simulink model "connecttoUDP_final"  (R2025a)
settings: Solver=ode4  StartTime=0.0  StopTime=inf  FixedStep=1/500  RelTol=1e-3  EnableMultiTasking=on
InitFcn:
  | home = [0.45; 0; 0.49];
  | pick = [0.3; 0; 0.3];
  | place = [-0.25; -0.25; 0.01];
  | waypoints = ...
  | [pick, pick,place ,place ,home]' ;
undefined symbols (not defined in the file): HIL, qc_get_step_size
libraries: quarc_library x19, simulink x3
(part 2 of 2)

== matlab function connecttoUDP_final/MATLAB Function ==
  settings: updateMethod=DISCRETE
  data: number output; p4 input; python_cmd input; gripper_cmd output; t input; is_visible input; gesto_to_int input; search_pos output
function [number, gripper_cmd, search_pos] = StateMachine(p4, python_cmd, t, is_visible, gesto_to_int)    
    
    persistent state
    persistent t_travel
    persistent t_visible
    persistent t_lost
    persistent t_gesture
    persistent current_y

    if isempty(state)
        state = 2; % 0 = Hunting the ball down, 1 = Going back to goal, 2 = Returning home and search
        t_travel = -1; % Putting a negative time stops the timer, used to find the travel time in each state mode
        t_visible = -1;
        t_lost = -1;
        t_gesture = -1;
        current_y = 0;
    end
    
    % Default safe position to output when not in State 2
    search_pos = [0.25; 0; 0.50];

    % --- Machine State Logic ---
    switch state
        
        case 0 % STATE 0: HUNTING THE BALL
            number = 1; % Connected on port 1 (xyz_mean)
            gripper_cmd = python_cmd; % The claw follows the camera
            
            % 1. CHECK IF BALL WAS CAUGHT
            if python_cmd == 1
                state = 3; 
                t_lost = -1; % Reset lost timer just in case
            end
            
            % 2. WATCHDOG TIMER: IF BALL IS LOST
            % If the camera goes blind, start the stopwatch before aborting
            if is_visible == 0
                if t_lost == -1
                    t_lost = t; % Start the lost stopwatch
                elseif (t - t_lost) >= 2.5 % Lost for more than 2.5 seconds
                    state = 2; % Go back to search mode
                    t_lost = -1; % Reset timer
                end
            else
                % Ball is visible, reset the stopwatch (Debounce)
                t_lost = -1; 
            end
            
        case 1 % STATE 1: DELIVERY (Advance in a straight line and release)
            number = 2; % We use port 2 to send a dynamic search_pos
            
            % 1. CALCULATE THE DYNAMIC TARGET POSITION
            % X was 0.25. We scale it by 2
            % Y is scaled by 2 in the exact same direction
            % Z is lowered to 0.40m
            target_x = 0.25 * 2; 
            target_y = current_y * 2;
            target_pos = [target_x; target_y; 0.40];
            
            % Send this position to the kinematics
            search_pos = target_pos; 
            
            % 2. IDENTIFY ARRIVAL AT TARGET
            distance_goal = norm(p4(1:3) - target_pos);
            
            if distance_goal < 0.05 && t_travel == -1
                t_travel = t; % Arrived! Start the delivery stopwatch  
            end
            
            % 3. DELIVERY TIMER LOGIC (Wait 1.0s -> Drop -> Wait 1s -> Leave)
            if t_travel ~= -1
                % If 4 seconds have passed (1.0s holding + 1s letting go)
                if (t - t_travel) >= 2.0
                    state = 2; % Mission accomplished! Return to Home/Search
                    t_travel = -1; % Reset timer
                    current_y = 0; % Reset joystick memory for next time
                    gripper_cmd = 1; % Claw still closed
                    
                % If 3 seconds have passed
                elseif (t - t_travel) >= 1.0 
                    gripper_cmd = 0; % OPEN CLAW (Drop the ball)
                    
                % If arrived but still waiting the initial 3 seconds
                else
                    gripper_cmd = 1; % KEEP CLAW CLOSED
                end
                
            else
                % Still traveling to the target
                gripper_cmd = 1; % Keep holding the ball tight
            end

        case 2 % STATE 2: SEARCH MODE (Go to alert position and sweep)
            number = 2; % Connected on port 2 (Search position)
            gripper_cmd = 0; % Keep claw open to not grab ghosts
            
            % 1. IDENTIFY ARRIVAL AT ALERT POSITION (Home)
            % Calculates distance to the base center position [0.25; 0; 0.50]
            distance_home = norm(p4(1:3) - [0.25; 0; 0.50]); 
            
            if distance_home < 0.05 && t_travel == -1
                t_travel = t; 
            end
            
            % 2. EXECUTE THE SINE WAVE SWEEP
            if t_travel == -1
                % Not there yet, keep target strictly at the center
                search_pos = [0.25; 0; 0.50];
            else
                % Start oscillating the Y axis                
                y_sweep = 0.25 * sin(0.30 * (t - t_travel));
                search_pos = [0.25; y_sweep; 0.50];
            end
            
            % 3. VERIFICATION BARRIER (DEBOUNCE LOGIC)
            if is_visible == 1
                if t_visible == -1
                    t_visible = t; % Ball spotted, start the stopwatch
                elseif (t - t_visible) >= 0.25 % Has it been consistently visible for 0.25 second
                    state = 0; % Barrier cleared! Transition to HUNTING
                    t_travel = -1; % Reset sweep timer
                    t_visible = -1; % Reset vision timer
                end
            else
                % False alarm or lost sight --> Reset stopwatch immediately
                t_visible = -1;
            end             

        case 3 % STATE 3: HOLD TARGET AND GESTURE JOYSTICK CONTROL
            number = 2; % Connect on port 2 (Search/Home position)
            gripper_cmd = 1; % KEEP CLAW CLOSED (Holding the ball)
            
            % 1. IDENTIFY ARRIVAL AT ALERT POSITION (Home)
            % Calculates distance to the base center position [0.25; 0; 0.50]
            distance_home = norm(p4(1:3) - [0.25; 0; 0.50]); 
            
            if distance_home < 0.05 && t_travel == -1
                t_travel = t; % Arrived! Unlock joystick control
                current_y = 0; % Reset joystick position to absolute center
            end
            
            % 2. EXECUTE THE JOYSTICK MOVEMENT BASED ON GESTURE
            if t_travel == -1
                % Not there yet, keep target strictly at the center
                search_pos = [0.25; 0; 0.50];
            else
                % Arrived at center. Now read the gesture to move!
                if gesto_to_int == 3 % RIGHT
                    current_y = current_y + 0.00010; % Move right smoothly
                    
                elseif gesto_to_int == 4 % LEFT
                    current_y = current_y - 0.00010; % Move left smoothly
                    
                end
                % Note: If gesture is NONE (0) or HAND (2), current_y is NOT modified. 
                % This creates the "freeze in place" smooth stop effect!
                
                % 3. SAFETY CLAMP (Mechanical Limits)
                % Prevent the arm from rotating beyond safe boundaries
                if current_y > 0.25
                    current_y = 0.25;
                elseif current_y < -0.25
                    current_y = -0.25;
                end
                
                % Output the accumulated position to the kinematics
                search_pos = [0.25; current_y; 0.50];
            end
            
            % 4. STOP GESTURE AND TRANSITION (With Debounce/Safety)
            % If the stop sign is shown AND the robot is already parked
            if gesto_to_int == 1 && t_travel ~= -1
                if t_gesture == -1
                    t_gesture = t; % AI saw STOP! Start the stopwatch
                elseif (t - t_gesture) >= 0.5 % Has it been a STOP for 0.5s?
                    state = 1; % Transition to the DELIVERY state
                    t_travel = -1; % Reset timer for the next state
                    t_gesture = -1; % Reset gesture timer
                end
            else
                % If it's not a STOP sign (false alarm or still moving), reset stopwatch
                t_gesture = -1; 
            end
            
        otherwise
            % Security against bugs 

            % 1. Fallback to the safest physical state
            state = 2; 
            number = 2; 
            search_pos = [0.25; 0; 0.50]; 
            gripper_cmd = 0; 
            
            % 2. Wipe all memory clean (Reset all timers)
            t_travel = -1;
            t_visible = -1;
            t_lost = -1;
            t_gesture = -1;
            current_y = 0;
    end
end

== matlab function connecttoUDP_final/TargetRangeLimiter ==
  data: p_obj_0 input; p_target output; R_max input
function p_target = radialClamp(p_obj_0, R_max)

eps_val = 1e-6;

norm_p = norm(p_obj_0);

if norm_p > R_max
    p_target = R_max * (p_obj_0 / (norm_p + eps_val));
else
    p_target = p_obj_0;
end

end

== matlab function connecttoUDP_final/MATLAB Function1 ==
  data: udp_data input size=[8 1]; t input size=1; X_filt output; Y_filt output; Z_filt output; gripper_cmd output; is_visible output; gesture_cmd output
function [X_filt, Y_filt, Z_filt, gripper_cmd, is_visible, gesture_cmd] = HybridSensorKalman(udp_data, t)
    % udp_data is a 7x1 vector from Python: 
    % [SensX, SensY, SensZ, PinhX, PinhY, PinhZ, FoundFlag]
    
    % Define the variables that will remember their values between Simulink steps
    persistent x_est P kf_initialized t_grip_start consecutive_outliers is_gripping

    % Initialize the Kalman Filter
    if isempty(kf_initialized)
        x_est = [0.2; 0.0; 0.3];  % Initial guess (Safe home position)
        P = eye(3) * 1.0;         % Initial uncertainty
        kf_initialized = true;
        t_grip_start = -1;        % Timer for gripper delay
        consecutive_outliers = 0; % Start counting outliers
        is_gripping = 0;          % Initialize grip state
    end

    % 1. Unpack UDP data and force double precision
    z_sens = double(udp_data(1:3));
    z_pinh = double(udp_data(4:6));
    found_flag = double(udp_data(7));
    gesture_cmd = double(udp_data(8));
    is_visible = found_flag;
    
    % Kalman tuning parameters (to be adjusted through trial and error)
    Q = eye(3) * 1e-6;   % Process Noise
    R_val = 8e-6;        % Measurement Variance

    % 2. Constant Position Kalman Prediction
    x_est = x_est;
    P = P + Q;

    % 3. Kalman Update (Sensor Fusion)
    if found_flag == 1
        % Determine depth
        depth = z_sens(3);
        if depth == 0 % Blind sensor scenario
            depth = z_pinh(3);
        end
        
        % Dynamic Confidence (Soft Switch)
        if depth < 0.25
            % Very close: Trust Pinhole 100%, Sensor 0%
            w_sens = 0.0; 
            w_pinh = 1.0;
        elseif depth > 0.35
            % Far away: Trust Sensor 100%, Pinhole 0%
            w_sens = 1.0; 
            w_pinh = 0.0;
        else
            % Transition Zone (25cm to 35cm): Cross-fade the signals
            w_sens = (depth - 0.25) / 0.10; 
            w_pinh = 1.0 - w_sens;
        end
        
        % Fused depth estimation
        z_fused = (w_sens * z_sens) + (w_pinh * z_pinh);
        
        % Outlier Detection (We check the Z depth specifically)
        distance_jump = abs(z_fused(3) - x_est(3));
        if distance_jump < 0.15
            % Normal Kalman update
            R = eye(3) * R_val;
            K = P / (P + R);
            x_est = x_est + K * (z_fused - x_est);
            P = (eye(3) - K) * P;

            consecutive_outliers = 0; % Reset counter

        else
            % Outlier detected
            consecutive_outliers = consecutive_outliers + 1;
            
            if consecutive_outliers > 3
                % Update position if not outlier
                x_est = z_fused;
                P = eye(3) * 1.0; % Reset uncertainty
                consecutive_outliers = 0;
            end
        end
    end

    % 4. Output filtered coordinates
    X_filt = x_est(1);
    Y_filt = x_est(2);
    Z_filt = x_est(3);

    % 5. Gripper Delay Logic
    dist_to_target = norm(x_est);

    if is_gripping == 0
        % Waiting for object
        if found_flag == 1 && dist_to_target <= 0.25
            if t_grip_start == -1
                t_grip_start = t; % Start timer
            elseif (t - t_grip_start) >= 0.75 
                is_gripping = 1; 
            end
        else
            t_grip_start = -1; % Reset timer if object moves away
        end
    else
        % Holding the object
        if gesture_cmd == 1
            is_gripping = 0;   % Release latch
            t_grip_start = -1; % Reset timer
        end
    end
    
    % Output the persistent state to the hardware
    gripper_cmd = is_gripping; 
end

== matlab function connecttoUDP_final/Champ cartésien ==
  data: p_current input; p_cmd output; p_target input; is_visible input
function  p_cmd= potentialFieldPlanner(p_current, p_target, is_visible)
% p_current : [3x1]
% p_target   : [3x1]
% is_visible: 0/1
% Ts        : pas de temps

%% Paramètres
k_att = 3.0;       % gain attractif
k_rep = 0.05;      % gain répulsif cylindre
v_max = 0.25;      % vitesse cartésienne max [m/s]

d0 = 0.15;         % rayon d'influence du cylindre
eps_norm = 1e-6;   % protection division par zéro

Ts=0.25

%% Si cible non visible : on garde la position actuelle
if is_visible == 0
    p_cmd = p_current;
    return;
end

%% --- Champ attractif ---
e = p_target - (p_current-[0.0;0.0;0.2]);
F_att = k_att * e;

%% --- Champ répulsif cylindre autour de la base ---
x = p_current(1);
y = p_current(2);
d = sqrt(x^2 + y^2);


if d < d0 && d > eps_norm
    n = [x; y; 0] / (d + eps_norm);
    F_rep = k_rep * (1/d - 1/d0) * (1/(d^2 + eps_norm)) * n;
else 
    F_rep=[0.0;0.0;0.0];
end

%% --- Champ total ---
F = F_att + F_rep;

%% --- Saturation smooth ---
F_norm = norm(F);

if F_norm > eps_norm
    v_cmd = v_max * tanh(F_norm / v_max) * (F / F_norm);
else
    v_cmd = [0;0;0];
end

%% --- Pas d'Euler ---
p_cmd = p_current + Ts * v_cmd;

end

== matlab function connecttoUDP_final/forward kinematics1 ==
  data: p3 output; R03 output; phi input; p4 output; R04 output; p_cam_0 output; p_obj_0 output; p_obj_cam input
function [p3, R03, p4, R04, p_cam_0,p_obj_0] = qarmForwardKinematics(phi,p_obj_cam)

%% QUANSER_ARM_FPK
% v 4.0 - 4th June 2020

% REFERENCE: 
% Chapter 3. Forward Kinematics
% Robot Dynamics and Control 
% Spong, Vidyasagar
% 1989

% INPUTS:
% phi     : Alternate joint angles vector 4 x 1

% OUTPUTS:
% p4      : End-effector frame {4} position vector expressed in base frame {0}
% R04     : rotation matrix from end-effector frame {4} to base frame {0}

%% Manipulator parameters:
L1 = 0.1400;
L2 = 0.3500;
L3 = 0.0500;
L4 = 0.2500;
L5 = 0.1500;

%% Alternate parameters
l1 = L1;
l2 = sqrt(L2^2 + L3^2);
l3 = L4 + L5;
beta = atan(L3/L2);

%% From phi space to theta space 
theta = phi;
theta(1) = phi(1);
theta(2) = phi(2) + beta - pi/2;
theta(3) = phi(3) - beta;
theta(4) = phi(4);

%% Transformation matrices for all frames:

% T{i-1}{i} = quanser_arm_DH(  a, alpha,  d,     theta );
        T01 = quanser_arm_DH(  0, -pi/2, l1,  theta(1) );
        T12 = quanser_arm_DH( l2,     0,  0,  theta(2) );
        T23 = quanser_arm_DH(  0, -pi/2,  0,  theta(3) );
        T34 = quanser_arm_DH(  0,     0, l3,  theta(4) );

        T02 = T01*T12;
        T03 = T02*T23;
        T04 = T03*T34;

%% Position of end-effector Transformation

% Extract the Position vector 
% p1   = T01(1:3,4);
% p2   = T02(1:3,4);
p3   = T03(1:3,4);
p4   = T04(1:3,4);

% Extract the Rotation matrix
% R01 = T01(1:3,1:3);
% R02 = T02(1:3,1:3);
R03 = T03(1:3,1:3);
R04 = T04(1:3,1:3);

d_tilde = 0.3; % distance entre P03 et la caméra (m)

% position de la caméra dans le frame de l'articulation 3
p_cam_3 = [0; 0; d_tilde]; 

% position de la caméra dans le frame global {0}
p_cam_0 = p3 + R03 * p_cam_3;

R_cam_3 = [ -1  0  0;
             0  1  0;
             0  0 -1 ];  % exemple si on inverse X et Z

R_cam_3 = [ 0  -1  0;
             1 0  0;
             0  0 1 ];  % exemple si on inverse X et Z

R_cam_0 = R03 * R_cam_3;  % rotation de la caméra dans le global

p_obj_0 = p_cam_0 + R_cam_0 * p_obj_cam;


end

function T = quanser_arm_DH(a,alpha,d,theta)

%% QUANSER_ARM_DH
% v 1.0 - 26th March 2019

% REFERENCE: 
% Chapter 3. Forward and Inverse Kinematics
% Robot Modeling and Control 
% Spong, Hutchinson, Vidyasagar
% 2006

% INPUTS:
% a       :   translation  : along : x_{i}   : from : z_{i-1} : to : z_{i}
% alpha   :      rotation  : about : x_{i}   : from : z_{i-1} : to : z_{i}
% d       :   translation  : along : z_{i-1} : from : x_{i-1} : to : x_{i}
% theta   :      rotation  : about : z_{i-1} : from : x_{i-1} : to : x_{i}
% NOTE: Standard DH Parameters

% OUTPUTS:
% T       : transformation                   : from :     {i} : to : {i-1}

%%
% Rotation Transformation about z axis by theta
T_R_z = [cos(theta) -sin(theta) 0 0;
         sin(theta)  cos(theta) 0 0;
                  0           0 1 0;
                  0           0 0 1];
     
% Translation Transformation along z axis by d
T_T_z = [1 0 0 0;
         0 1 0 0;
         0 0 1 d;
         0 0 0 1];

% Translation Transformation along x axis by a
T_T_x = [1 0 0 a;
         0 1 0 0;
         0 0 1 0;
         0 0 0 1];

% Rotation Transformation about x axis by alpha
T_R_x = [1          0           0 0;
         0 cos(alpha) -sin(alpha) 0;
         0 sin(alpha)  cos(alpha) 0;
         0          0           0 1];

% For a transformation FROM frame {i} TO frame {i-1}: A
T = T_R_z*T_T_z*T_T_x*T_R_x;

end

== matlab function connecttoUDP_final/forward kinematics2 ==
  data: xyz input; xyz_mean output
function xyz_mean = mean_xyz_1s(xyz)
% xyz : [3x1] ou [1x3]
% xyz_mean : [3x1] moyenne sur 1 seconde

    %#codegen

    % PARAMÈTRES
    N = 1;   % nombre d'échantillons pour 1 seconde (Ts = 0.01s)

    % PERSISTANTS À TAILLE FIXE
    persistent buffer index count

    if isempty(buffer)
        buffer = zeros(3, N);
        index  = 1;
        count  = 0;
    end

    % Forcer vecteur colonne
    xyz = xyz(:);

    % Stockage circulaire
    buffer(:, index) = xyz;

    index = index + 1;
    if index > N
        index = 1;
    end

    if count < N
        count = count + 1;
    end

    % Moyenne
    xyz_mean = sum(buffer(:,1:count), 2) / count;

end

== matlab function connecttoUDP_final/forward kinematics ==
  data: phi input; p4 output; R04 output
function [p4, R04] = qarmForwardKinematics(phi)

%% QUANSER_ARM_FPK
% v 4.0 - 4th June 2020

% REFERENCE: 
% Chapter 3. Forward Kinematics
% Robot Dynamics and Control 
% Spong, Vidyasagar
% 1989

% INPUTS:
% phi     : Alternate joint angles vector 4 x 1

% OUTPUTS:
% p4      : End-effector frame {4} position vector expressed in base frame {0}
% R04     : rotation matrix from end-effector frame {4} to base frame {0}

%% Manipulator parameters:
L1 = 0.1400;
L2 = 0.3500;
L3 = 0.0500;
L4 = 0.2500;
L5 = 0.1500;

%% Alternate parameters
l1 = L1;
l2 = sqrt(L2^2 + L3^2);
l3 = L4 + L5;
beta = atan(L3/L2);

%% From phi space to theta space 
theta = phi;
theta(1) = phi(1);
theta(2) = phi(2) + beta - pi/2;
theta(3) = phi(3) - beta;
theta(4) = phi(4);

%% Transformation matrices for all frames:

% T{i-1}{i} = quanser_arm_DH(  a, alpha,  d,     theta );
        T01 = quanser_arm_DH(  0, -pi/2, l1,  theta(1) );
        T12 = quanser_arm_DH( l2,     0,  0,  theta(2) );
        T23 = quanser_arm_DH(  0, -pi/2,  0,  theta(3) );
        T34 = quanser_arm_DH(  0,     0, l3,  theta(4) );

        T02 = T01*T12;
        T03 = T02*T23;
        T04 = T03*T34;

%% Position of end-effector Transformation

% Extract the Position vector 
% p1   = T01(1:3,4);
% p2   = T02(1:3,4);
% p3   = T03(1:3,4);
p4   = T04(1:3,4);

% Extract the Rotation matrix
% R01 = T01(1:3,1:3);
% R02 = T02(1:3,1:3);
% R03 = T03(1:3,1:3);
R04 = T04(1:3,1:3);

end

function T = quanser_arm_DH(a,alpha,d,theta)

%% QUANSER_ARM_DH
% v 1.0 - 26th March 2019

% REFERENCE: 
% Chapter 3. Forward and Inverse Kinematics
% Robot Modeling and Control 
% Spong, Hutchinson, Vidyasagar
% 2006

% INPUTS:
% a       :   translation  : along : x_{i}   : from : z_{i-1} : to : z_{i}
% alpha   :      rotation  : about : x_{i}   : from : z_{i-1} : to : z_{i}
% d       :   translation  : along : z_{i-1} : from : x_{i-1} : to : x_{i}
% theta   :      rotation  : about : z_{i-1} : from : x_{i-1} : to : x_{i}
% NOTE: Standard DH Parameters

% OUTPUTS:
% T       : transformation                   : from :     {i} : to : {i-1}

%%
% Rotation Transformation about z axis by theta
T_R_z = [cos(theta) -sin(theta) 0 0;
         sin(theta)  cos(theta) 0 0;
                  0           0 1 0;
                  0           0 0 1];
     
% Translation Transformation along z axis by d
T_T_z = [1 0 0 0;
         0 1 0 0;
         0 0 1 d;
         0 0 0 1];

% Translation Transformation along x axis by a
T_T_x = [1 0 0 a;
         0 1 0 0;
         0 0 1 0;
         0 0 0 1];

% Rotation Transformation about x axis by alpha
T_R_x = [1          0           0 0;
         0 cos(alpha) -sin(alpha) 0;
         0 sin(alpha)  cos(alpha) 0;
         0          0           0 1];

% For a transformation FROM frame {i} TO frame {i-1}: A
T = T_R_z*T_T_z*T_T_x*T_R_x;

end

== matlab function connecttoUDP_final/inverse kinematics ==
  data: p input; gamma input; phi_optimal output; phi_prev input
function phi_optimal = qarmInverseKinematics(p, gamma, phi_prev)
%% QARM Inverse Kinematics with singularity avoidance
% Gère :
% 1) singularité "effecteur au-dessus de la base" via exclusion cylindrique
% 2) singularité de l'articulation 3 : theta3 = +/- 90 deg
%
% INPUTS:
%   p        : position [x;y;z] en m
%   gamma    : rotation poignet (rad)
%   phi_prev : configuration précédente [4x1] en rad
%
% OUTPUT:
%   phi_optimal : configuration atteignable [4x1] rad

%% Paramètres du manipulateur
L1 = 0.1400; 
L2 = 0.3500; 
L3 = 0.0500; 
L4 = 0.2500; 
L5 = 0.1500;

beta = atan(L3/L2);

lambda1 = L1;
lambda2 = sqrt(L2^2 + L3^2);
lambda3 = L4 + L5;

%% Paramètres d'évitement des singularités A ADAPTER PAS ENCORE DE TEST FAIT SUR ROBOT 
R_MIN = 0.08;                 % rayon mini du cylindre d'exclusion (m)
EPS_DEN = 1e-6;               % protection divisions
EPS_COST = 1e-4;              % protection coût singularité

W_CONT = 1.0;                 % poids continuité avec phi_prev
W_SING_THETA3 = 0.25;         % poids singularité theta3 = +/- pi/2
W_LIMIT = 0.05;               % petit poids pour éloigner des butées

%% --- 1) Exclusion cylindrique autour de la base ---
% On évite une zone cylindrique autour de la base (le bras se bloque quand
% il y entre).
% Ici, on régularise directement la cible cartésienne.
p_reg = p;
r = hypot(p(1), p(2));

if r < R_MIN
    if r > EPS_DEN
        p_reg(1) = p(1) * R_MIN / r;
        p_reg(2) = p(2) * R_MIN / r;
    else
        % Si on est exactement sur l'axe, on prend la direction de la base précédente
        base_dir = phi_prev(1);
        p_reg(1) = R_MIN * cos(base_dir);
        p_reg(2) = R_MIN * sin(base_dir);
    end
end

%% Initialisation
theta = zeros(4,4);
phi   = zeros(4,4);

%% --- Calcul theta2 / theta3 ---
A = lambda2; 
C = -lambda3; 
H = lambda1 - p_reg(3);

D1 = -hypot(p_reg(1), p_reg(2)); 
D2 =  hypot(p_reg(1), p_reg(2));

F1 = (D1^2 + H^2 - A^2 - C^2)/(2*A);
F2 = (D2^2 + H^2 - A^2 - C^2)/(2*A);

% Si racine négative, saturation
if C^2 - F1^2 < 0
    warning('Position non atteignable pour solution 1/2 : saturation');
    theta(3,1) = sign(C)*pi/2;
    theta(3,2) = sign(C)*pi/2;
else
    theta(3,1) = 2*atan2(C + sqrt(C^2 - F1^2), F1);
    theta(3,2) = 2*atan2(C - sqrt(C^2 - F1^2), F1);
end

if C^2 - F2^2 < 0
    warning('Position non atteignable pour solution 3/4 : saturation');
    theta(3,3) = sign(C)*pi/2;
    theta(3,4) = sign(C)*pi/2;
else
    theta(3,3) = 2*atan2(C + sqrt(C^2 - F2^2), F2);
    theta(3,4) = 2*atan2(C - sqrt(C^2 - F2^2), F2);
end

%% --- Calcul theta2 ---
for i = 1:4
    D = D1; 
    if i > 2
        D = D2; 
    end

    M = A + C*sin(theta(3,i));
    N = -C*cos(theta(3,i));

    if abs(M) < EPS_DEN
        M = sign_nonzero(M) * EPS_DEN;
    end

    cos_term = (D*M + H*N)/(M^2 + N^2);
    sin_term = (H - N*cos_term)/M;
    theta(2,i) = atan2(sin_term, cos_term);
end

%% --- Calcul theta1 ---
for i = 1:4
    denom = lambda2*cos(theta(2,i)) - lambda3*sin(theta(2,i)+theta(3,i));
    if abs(denom) < EPS_DEN
        denom = sign_nonzero(denom) * EPS_DEN;
    end
    theta(1,i) = atan2(p_reg(2)/denom, p_reg(1)/denom);
end

%% --- Remap vers angles QARM ---
phi(1,:) = theta(1,:);
phi(2,:) = theta(2,:) - beta + pi/2;
phi(3,:) = theta(3,:) + beta;
phi(4,:) = gamma;

phi = wrapToPiLocal(phi);

%% --- Saturation des limites ---
for i = 1:4
    phi(:,i) = saturate_joint_limits(phi(:,i));
end

%% --- Choix de la meilleure solution avec pénalisation singularités ---
phi_optimal = phi(:,1);
best_cost = candidate_cost(phi(:,1), theta(:,1), phi_prev, R_MIN, r, W_CONT, W_SING_THETA3, W_LIMIT, EPS_COST);

for i = 2:4
    current_cost = candidate_cost(phi(:,i), theta(:,i), phi_prev, R_MIN, r, W_CONT, W_SING_THETA3, W_LIMIT, EPS_COST);
    if isnan(current_cost)
        continue;
    end
    if current_cost < best_cost
        phi_optimal = phi(:,i);
        best_cost = current_cost;
    end
end

if any(isnan(phi_optimal))
    warning('NaN détecté dans phi_optimal, retour à phi_prev');
    phi_optimal = phi_prev;
end

end

%% ===================== COST FUNCTION =====================
function J = candidate_cost(phi_i, theta_i, phi_prev, R_MIN, r_raw, W_CONT, W_SING_THETA3, W_LIMIT, EPS_COST)

    % 1) Continuité avec la configuration précédente
    dphi = wrapToPiLocal(phi_i - phi_prev);
    J_cont = norm(dphi);

    % 2) Pénalisation singularité theta3 = +/- 90 deg
    % Rapport : singularité quand theta3 = +/- pi/2
    d1 = abs(wrapToPiLocal(theta_i(3) - pi/2));
    d2 = abs(wrapToPiLocal(theta_i(3) + pi/2));
    J_sing_theta3 = 1/(d1^2 + EPS_COST) + 1/(d2^2 + EPS_COST);

    % 3) Petite pénalisation si on est près des butées
    J_limits = joint_limit_barrier(phi_i, EPS_COST);

    % 4) Pénalisation brute si la cible originale était trop près de l'axe base
    % (même si régularisée ensuite)
    if r_raw < R_MIN
        J_base = 1 + 10*(R_MIN - r_raw)^2;
    else
        J_base = 0;
    end

    J = W_CONT * J_cont + ...
        W_SING_THETA3 * J_sing_theta3 + ...
        W_LIMIT * J_limits + ...
        J_base;
end

%% ===================== JOINT LIMITS =====================
function phi_sat = saturate_joint_limits(phi)
% C'est les mêmes limites qu'avant mais ça peut être intéressant à régler 
limits = [
    -170  170;
    -80    80;
    -95    75;
    -160  160
] * pi/180;

phi_sat = phi;
for i = 1:4
    if phi(i) < limits(i,1)
        phi_sat(i) = limits(i,1);
    end
    if phi(i) > limits(i,2)
        phi_sat(i) = limits(i,2);
    end
end
end

function J = joint_limit_barrier(phi, eps_cost)
limits = [
    -170  170;
    -80    80;
    -95    75;
    -160  160
] * pi/180;

J = 0;
for k = 1:4
    dmin = abs(phi(k) - limits(k,1));
    dmax = abs(limits(k,2) - phi(k));
    J = J + 1/(dmin^2 + eps_cost) + 1/(dmax^2 + eps_cost);
end
end

%% ===================== HELPERS =====================
function y = wrapToPiLocal(x)
y = mod(x + pi, 2*pi) - pi;
end

function s = sign_nonzero(x)
if x >= 0
    s = 1;
else
    s = -1;
end
end

== matlab function connecttoUDP_final/differential kinematics ==
  data: phi input; J output
function J   = qarmDifferentialKinematics(phi)

%% QUANSER_ARM_FDK
% v 1.0 - 13th August 2020

% REFERENCE: 
% Chapter 5. Velocity Kinematics
% Robot Dynamics and Control 
% Spong, Vidyasagar
% 1989

% INPUTS:
% phi     : Alternate joint angles vector 4 x 1

% OUTPUTS:
% p4      : End-effector frame {4} position vector expressed in base frame {0}
% R04     : rotation matrix from end-effector frame {4} to base frame {0}

%% Manipulator parameters:
L1 = 0.1400;
L2 = 0.3500;
L3 = 0.0500;
L4 = 0.2500;
L5 = 0.1500;

%% Alternate parameters
l1 = L1;
l2 = sqrt(L2^2 + L3^2);
l3 = L4 + L5;
beta = atan(L3/L2);

%% From phi space to theta space 
theta = phi;
theta(1) = phi(1);
theta(2) = phi(2) + beta - pi/2;
theta(3) = phi(3) - beta;
theta(4) = phi(4);

%% Precompute sines and cosines
c1 = cos(theta(1)); s1 = sin(theta(1));
c2 = cos(theta(2)); s2 = sin(theta(2));
c23 = cos(theta(2) + theta(3)); s23 = sin(theta(2) + theta(3));

%% Jacobian term definition:

J = eye(4);
J(1,1) = -l2 * s1 * c2 + l3 * s1 * s23;
J(1,2) = -l2 * c1 * s2 - l3 * c1 * c23;
J(1,3) = -l3 * c1 * c23;
J(1,4) = 0;

J(2,1) =  l2 * c1 * c2 - l3 * c1 * s23;
J(2,2) = -l2 * s1 * s2 - l3 * s1 * c23;
J(2,3) = -l3 * s1 * c23;
J(2,4) = 0;

J(3,1) =  0;
J(3,2) = -l2 * c2 + l3 * s23;
J(3,3) =  l3 * s23;
J(3,4) = 0;

J(4,1) =  0;
J(4,2) =  0;
J(4,3) =  0;
J(4,4) =  1;

end

== matlab function connecttoUDP_final/forward kinematics - measurement ==
  data: phi input; p4 output; R04 output
function [p4, R04] = qarmForwardKinematics(phi)

%% QUANSER_ARM_FPK
% v 4.0 - 4th June 2020

% REFERENCE: 
% Chapter 3. Forward Kinematics
% Robot Dynamics and Control 
% Spong, Vidyasagar
% 1989

% INPUTS:
% phi     : Alternate joint angles vector 4 x 1

% OUTPUTS:
% p4      : End-effector frame {4} position vector expressed in base frame {0}
% R04     : rotation matrix from end-effector frame {4} to base frame {0}

%% Manipulator parameters:
L1 = 0.1400;
L2 = 0.3500;
L3 = 0.0500;
L4 = 0.2500;
L5 = 0.1500;

%% Alternate parameters
l1 = L1;
l2 = sqrt(L2^2 + L3^2);
l3 = L4 + L5;
beta = atan(L3/L2);

%% From phi space to theta space 
theta = phi;
theta(1) = phi(1);
theta(2) = phi(2) + beta - pi/2;
theta(3) = phi(3) - beta;
theta(4) = phi(4);

%% Transformation matrices for all frames:

% T{i-1}{i} = quanser_arm_DH(  a, alpha,  d,     theta );
        T01 = quanser_arm_DH(  0, -pi/2, l1,  theta(1) );
        T12 = quanser_arm_DH( l2,     0,  0,  theta(2) );
        T23 = quanser_arm_DH(  0, -pi/2,  0,  theta(3) );
        T34 = quanser_arm_DH(  0,     0, l3,  theta(4) );

        T02 = T01*T12;
        T03 = T02*T23;
        T04 = T03*T34;

%% Position of end-effector Transformation

% Extract the Position vector 
% p1   = T01(1:3,4);
% p2   = T02(1:3,4);
% p3   = T03(1:3,4);
p4   = T04(1:3,4);

% Extract the Rotation matrix
% R01 = T01(1:3,1:3);
% R02 = T02(1:3,1:3);
% R03 = T03(1:3,1:3);
R04 = T04(1:3,1:3);

end

function T = quanser_arm_DH(a,alpha,d,theta)

%% QUANSER_ARM_DH
% v 1.0 - 26th March 2019

% REFERENCE: 
% Chapter 3. Forward and Inverse Kinematics
% Robot Modeling and Control 
% Spong, Hutchinson, Vidyasagar
% 2006

% INPUTS:
% a       :   translation  : along : x_{i}   : from : z_{i-1} : to : z_{i}
% alpha   :      rotation  : about : x_{i}   : from : z_{i-1} : to : z_{i}
% d       :   translation  : along : z_{i-1} : from : x_{i-1} : to : x_{i}
% theta   :      rotation  : about : z_{i-1} : from : x_{i-1} : to : x_{i}
% NOTE: Standard DH Parameters

% OUTPUTS:
% T       : transformation                   : from :     {i} : to : {i-1}

%%
% Rotation Transformation about z axis by theta
T_R_z = [cos(theta) -sin(theta) 0 0;
         sin(theta)  cos(theta) 0 0;
                  0           0 1 0;
                  0           0 0 1];
     
% Translation Transformation along z axis by d
T_T_z = [1 0 0 0;
         0 1 0 0;
         0 0 1 d;
         0 0 0 1];

% Translation Transformation along x axis by a
T_T_x = [1 0 0 a;
         0 1 0 0;
         0 0 1 0;
         0 0 0 1];

% Rotation Transformation about x axis by alpha
T_R_x = [1          0           0 0;
         0 cos(alpha) -sin(alpha) 0;
         0 sin(alpha)  cos(alpha) 0;
         0          0           0 1];

% For a transformation FROM frame {i} TO frame {i-1}: A
T = T_R_z*T_T_z*T_T_x*T_R_x;

end

== matlab function connecttoUDP_final/forward kinematics3 ==
  data: phi input; p4 output; R04 output
function [p4, R04] = qarmForwardKinematics(phi)

%% QUANSER_ARM_FPK
% v 4.0 - 4th June 2020

% REFERENCE: 
% Chapter 3. Forward Kinematics
% Robot Dynamics and Control 
% Spong, Vidyasagar
% 1989

% INPUTS:
% phi     : Alternate joint angles vector 4 x 1

% OUTPUTS:
% p4      : End-effector frame {4} position vector expressed in base frame {0}
% R04     : rotation matrix from end-effector frame {4} to base frame {0}

%% Manipulator parameters:
L1 = 0.1400;
L2 = 0.3500;
L3 = 0.0500;
L4 = 0.2500;
L5 = 0.1500;

%% Alternate parameters
l1 = L1;
l2 = sqrt(L2^2 + L3^2);
l3 = L4 + L5;
beta = atan(L3/L2);

%% From phi space to theta space 
theta = phi;
theta(1) = phi(1);
theta(2) = phi(2) + beta - pi/2;
theta(3) = phi(3) - beta;
theta(4) = phi(4);

%% Transformation matrices for all frames:

% T{i-1}{i} = quanser_arm_DH(  a, alpha,  d,     theta );
        T01 = quanser_arm_DH(  0, -pi/2, l1,  theta(1) );
        T12 = quanser_arm_DH( l2,     0,  0,  theta(2) );
        T23 = quanser_arm_DH(  0, -pi/2,  0,  theta(3) );
        T34 = quanser_arm_DH(  0,     0, l3,  theta(4) );

        T02 = T01*T12;
        T03 = T02*T23;
        T04 = T03*T34;

%% Position of end-effector Transformation

% Extract the Position vector 
% p1   = T01(1:3,4);
% p2   = T02(1:3,4);
% p3   = T03(1:3,4);
p4   = T04(1:3,4);

% Extract the Rotation matrix
% R01 = T01(1:3,1:3);
% R02 = T02(1:3,1:3);
% R03 = T03(1:3,1:3);
R04 = T04(1:3,1:3);

end

function T = quanser_arm_DH(a,alpha,d,theta)

%% QUANSER_ARM_DH
% v 1.0 - 26th March 2019

% REFERENCE: 
% Chapter 3. Forward and Inverse Kinematics
% Robot Modeling and Control 
% Spong, Hutchinson, Vidyasagar
% 2006

% INPUTS:
% a       :   translation  : along : x_{i}   : from : z_{i-1} : to : z_{i}
% alpha   :      rotation  : about : x_{i}   : from : z_{i-1} : to : z_{i}
% d       :   translation  : along : z_{i-1} : from : x_{i-1} : to : x_{i}
% theta   :      rotation  : about : z_{i-1} : from : x_{i-1} : to : x_{i}
% NOTE: Standard DH Parameters

% OUTPUTS:
% T       : transformation                   : from :     {i} : to : {i-1}

%%
% Rotation Transformation about z axis by theta
T_R_z = [cos(theta) -sin(theta) 0 0;
         sin(theta)  cos(theta) 0 0;
                  0           0 1 0;
                  0           0 0 1];
     
% Translation Transformation along z axis by d
T_T_z = [1 0 0 0;
         0 1 0 0;
         0 0 1 d;
         0 0 0 1];

% Translation Transformation along x axis by a
T_T_x = [1 0 0 a;
         0 1 0 0;
         0 0 1 0;
         0 0 0 1];

% Rotation Transformation about x axis by alpha
T_R_x = [1          0           0 0;
         0 cos(alpha) -sin(alpha) 0;
         0 sin(alpha)  cos(alpha) 0;
         0          0           0 1];

% For a transformation FROM frame {i} TO frame {i-1}: A
T = T_R_z*T_T_z*T_T_x*T_R_x;

end

== matlab function connecttoUDP_final/forward kinematics - setpoint ==
  data: phi input; p4 output; R04 output
function [p4, R04] = qarmForwardKinematics(phi)

%% QUANSER_ARM_FPK
% v 4.0 - 4th June 2020

% REFERENCE: 
% Chapter 3. Forward Kinematics
% Robot Dynamics and Control 
% Spong, Vidyasagar
% 1989

% INPUTS:
% phi     : Alternate joint angles vector 4 x 1

% OUTPUTS:
% p4      : End-effector frame {4} position vector expressed in base frame {0}
% R04     : rotation matrix from end-effector frame {4} to base frame {0}

%% Manipulator parameters:
L1 = 0.1400;
L2 = 0.3500;
L3 = 0.0500;
L4 = 0.2500;
L5 = 0.1500;

%% Alternate parameters
l1 = L1;
l2 = sqrt(L2^2 + L3^2);
l3 = L4 + L5;
beta = atan(L3/L2);

%% From phi space to theta space 
theta = phi;
theta(1) = phi(1);
theta(2) = phi(2) + beta - pi/2;
theta(3) = phi(3) - beta;
theta(4) = phi(4);

%% Transformation matrices for all frames:

% T{i-1}{i} = quanser_arm_DH(  a, alpha,  d,     theta );
        T01 = quanser_arm_DH(  0, -pi/2, l1,  theta(1) );
        T12 = quanser_arm_DH( l2,     0,  0,  theta(2) );
        T23 = quanser_arm_DH(  0, -pi/2,  0,  theta(3) );
        T34 = quanser_arm_DH(  0,     0, l3,  theta(4) );

        T02 = T01*T12;
        T03 = T02*T23;
        T04 = T03*T34;

%% Position of end-effector Transformation

% Extract the Position vector 
% p1   = T01(1:3,4);
% p2   = T02(1:3,4);
% p3   = T03(1:3,4);
p4   = T04(1:3,4);

% Extract the Rotation matrix
% R01 = T01(1:3,1:3);
% R02 = T02(1:3,1:3);
% R03 = T03(1:3,1:3);
R04 = T04(1:3,1:3);

end

function T = quanser_arm_DH(a,alpha,d,theta)

%% QUANSER_ARM_DH
% v 1.0 - 26th March 2019

% REFERENCE: 
% Chapter 3. Forward and Inverse Kinematics
% Robot Modeling and Control 
% Spong, Hutchinson, Vidyasagar
% 2006

% INPUTS:
% a       :   translation  : along : x_{i}   : from : z_{i-1} : to : z_{i}
% alpha   :      rotation  : about : x_{i}   : from : z_{i-1} : to : z_{i}
% d       :   translation  : along : z_{i-1} : from : x_{i-1} : to : x_{i}
% theta   :      rotation  : about : z_{i-1} : from : x_{i-1} : to : x_{i}
% NOTE: Standard DH Parameters

% OUTPUTS:
% T       : transformation                   : from :     {i} : to : {i-1}

%%
% Rotation Transformation about z axis by theta
T_R_z = [cos(theta) -sin(theta) 0 0;
         sin(theta)  cos(theta) 0 0;
                  0           0 1 0;
                  0           0 0 1];
     
% Translation Transformation along z axis by d
T_T_z = [1 0 0 0;
         0 1 0 0;
         0 0 1 d;
         0 0 0 1];

% Translation Transformation along x axis by a
T_T_x = [1 0 0 a;
         0 1 0 0;
         0 0 1 0;
         0 0 0 1];

% Rotation Transformation about x axis by alpha
T_R_x = [1          0           0 0;
         0 cos(alpha) -sin(alpha) 0;
         0 sin(alpha)  cos(alpha) 0;
         0          0           0 1];

% For a transformation FROM frame {i} TO frame {i-1}: A
T = T_R_z*T_T_z*T_T_x*T_R_x;

end
